simulink model "sim_cassie"  (R2017b)
settings: Solver=VariableStepAuto  StartTime=0.0  StopTime=0.70  RelTol=1e-3
InitFcn:
  | stance_leg = 1;
  | initial_speed = [0.0, 0]; % [vx0, vy0];
  | 
  | % Load gait parameter library
  | load('gaitLib_interp');
  | gait_param = param_lib(initial_speed(1), stance_leg, interp_lib);
  | 
  | x0 = gait_param.x0;
  | 
  | control_rate = 4000; % hz
values from neighbouring files (symbols this model uses):
  interp_lib = []    [GaitParams.m]
settings Model: Creator=jreher  LastModifiedBy=jreher
settings DebuggingCC: AlgebraicLoopMsg=none

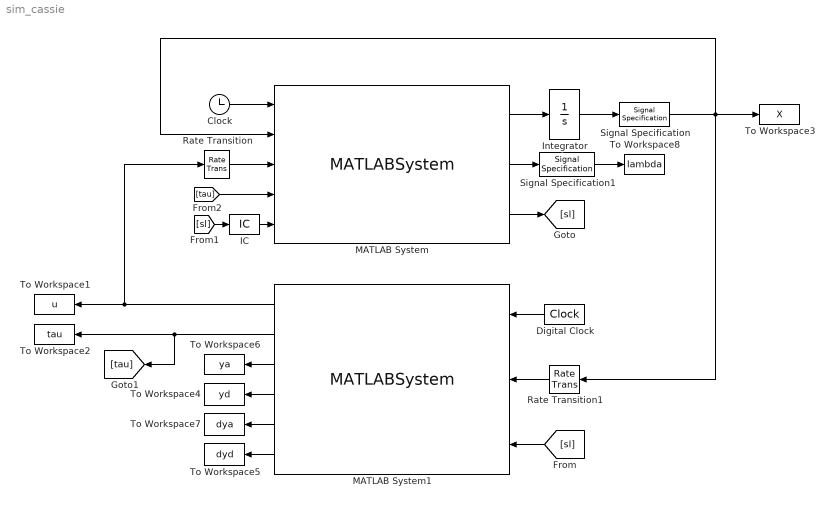
== system sim_cassie ==
  Clock : Clock
  Digital Clock : DigitalClock  SampleTime=1/control_rate
  IC : InitialCondition  Value=stance_leg
  Integrator : Integrator  InitialCondition=x0
  MATLAB System : MATLABSystem  System=CassieDynamics  SimulateUsing=Interpreted execution
      mask Type: CassieDynamics
      mask Display:
      | disp('CassieDynamics');
      | port_label('input',1,'t');
      | port_label('input',2,'X');
      | port_label('input',3,'u');
      | port_label('input',4,'tau');
      | port_label('input',5,'stance');
      | port_label('output',1,'dX');
      | port_label('output',2,'lambda');
      | port_label('output',3,'stance');
  MATLAB System1 : MATLABSystem  System=CassieQPcontroller  SimulateUsing=Interpreted execution
      mask Type: CassieQPcontroller
      mask Display:
      | disp('CassieQPcontroller');
      | port_label('input',1,'t');
      | port_label('input',2,'X');
      | port_label('input',3,'stance');
      | port_label('output',1,'u');
      | port_label('output',2,'tau');
      | port_label('output',3,'ya');
      | port_label('output',4,'yd');
      | port_label('output',5,'dya');
      | port_label('output',6,'dyd');
  Rate Transition : RateTransition
  Rate Transition1 : RateTransition  OutPortSampleTime=1/control_rate
  Signal Specification : SignalSpecification  Dimensions=44
  Signal Specification1 : SignalSpecification  Dimensions=9
  To Workspace1 : ToWorkspace  VariableName=u  SaveFormat=Timeseries  SampleTime=-1
  To Workspace2 : ToWorkspace  VariableName=tau  SaveFormat=Timeseries  SampleTime=-1
  To Workspace3 : ToWorkspace  VariableName=X  SaveFormat=Timeseries  SampleTime=-1
  To Workspace4 : ToWorkspace  VariableName=yd  SaveFormat=Timeseries  SampleTime=-1
  To Workspace5 : ToWorkspace  VariableName=dyd  SaveFormat=Timeseries  SampleTime=-1
  To Workspace6 : ToWorkspace  VariableName=ya  SaveFormat=Timeseries  SampleTime=-1
  To Workspace7 : ToWorkspace  VariableName=dya  SaveFormat=Timeseries  SampleTime=-1
  To Workspace8 : ToWorkspace  VariableName=lambda  SaveFormat=Timeseries  SampleTime=-1
  wires:
  MATLAB System/1 -> Integrator/1
  Integrator/1 -> Signal Specification/1
  Digital Clock/1 -> MATLAB System1/1
  Clock/1 -> MATLAB System/1
  Signal Specification/1 -> To Workspace3/1, Rate Transition1/1, MATLAB System/2
  MATLAB System/2 -> Signal Specification1/1
  Rate Transition1/1 -> MATLAB System1/2
  Signal Specification1/1 -> To Workspace8/1
  MATLAB System/3 -> [sl]
  [sl] -> MATLAB System1/3
  [sl] -> IC/1
  MATLAB System1/2 -> [tau], To Workspace2/1
  MATLAB System1/3 -> To Workspace6/1
  MATLAB System1/4 -> To Workspace4/1
  MATLAB System1/5 -> To Workspace7/1
  MATLAB System1/6 -> To Workspace5/1
  Rate Transition/1 -> MATLAB System/3
  MATLAB System1/1 -> To Workspace1/1, Rate Transition/1
  IC/1 -> MATLAB System/5
  [tau] -> MATLAB System/4
